simulink model "c8mfpid"  (R2019b)
settings: Solver=VariableStepAuto  StartTime=0.0  StopTime=20  RelTol=1e-11
PreLoadFcn:
  | s=fotf('s'); G=1/(0.8*s^2.2+0.5*s^0.9+1);
  | ww=[1e-4, 1e4]; N=11;
libraries: cstblocks x2
settings Model: Creator=xuedi  LastModifiedBy=xuedi
settings DataIOCC: SaveFormat=Array  ReturnWorkspaceOutputs=off
settings DebuggingCC: UnconnectedInputMsg=none  UnconnectedOutputMsg=none  UnconnectedLineMsg=none  SFMachineParentedDataDiag=error

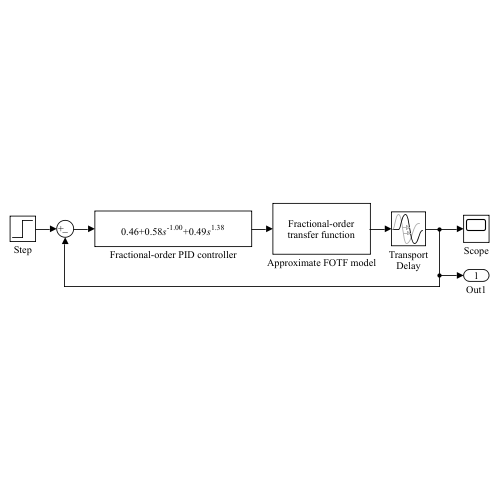
[thumbnail: Simulink's stored preview of the top-level diagram]
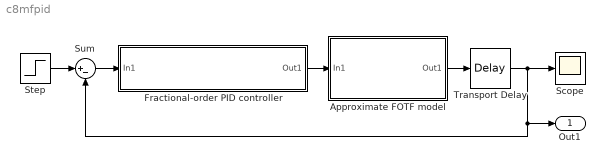
== system c8mfpid ==
  Approximate FOTF model : Subsystem  mask{na=[2.2 0.9 0], a=[0.8 0.5 1], nb=0, b=1, ww=ww, N=N, kFilter=Oustaloup filter, T=0}
      mask prompts: na "Orders of the denominator"; a "Coefficients of the denominator"; nb "Orders of the numerator"; b "Coefficients of the numerator"; ww "Interested frequency range [wb wh]"; N "Filter order"; kFilter "Types of the filter"; T "Delay constant T"
      mask init:
      | if isa(na,'fotf'), G=na; 
      |    else
      |       if length(na)~=length(a)
      |          errordlg('Error','Mismatch on the denominator'), 
      |       end
      |       if length(b)~=length(nb)
      |          errordlg('Error','Mismatch on the numerator'), 
      |       end
      |       G=fotf(a,na,b,nb);
      |    end
      |    switch kFilter
      |       case 1, str='ousta_fod'; 
      |       case 2, str='new_fod'; 
      |       case 3, str='matsude_fod';
      |    end
      |    wb=ww(1); wh=ww(2); G1=high_order(G,str,wb,wh,N); 
      |    G1.ioDelay=T;
      mask TypeOptions kFilter: Oustaloup filter | Modified Oustaloup filter
      mask Display: disp('Fractional-order\ntransfer function')
  Fractional-order PID controller : Subsystem  mask{Kp=0.45966, II=[0.5761 0.99627], DD=[0.49337 1.3792], N=N, ww=ww, kFilter=Oustaloup filter}
      mask prompts: Kp "Proportional Kp"; II "Integral [Ki lam]"; DD "Differentiation [Kd mu]"; N "Filter order"; ww "Interested frequency range [wb wh]"; kFilter "Types of the filter"
      mask init:
      | if isa(Kp,'fotf'), a=Kp;
      |       lam=a.den.na; mu=a.num.na; mu=mu(1)-lam; b=a.num.a; Kd=b(1); Kp=b(2); Ki=b(3);
      |    else, II=[II 1]; DD=[DD 1]; Ki=II(1); lam=II(2); Kd=DD(1); mu=DD(2); end
      |    s=tf('s'); 
      |    sI=ousta_fod(1-lam,N,ww(1),ww(2)); sD=ousta_fod(mu,N,ww(1),ww(2));
      |    Gc=Kp+Ki*sI/s+Kd*sD;
      |    if abs(Ki)>0, sI=[sprintf('%.2f',Ki),'{\its}^{' sprintf('%.2f',-lam), '}']; end
      |    if abs(Kd)>0, sD=[sprintf('%.2f',Kd),'{\its}^{' sprintf('%.2f',mu), '}']; end
      |    str=sprintf('%.2f',Kp);
      |    if abs(Ki)>0, if sI(1)~='-', sI=['+' sI]; end, str=[str,sI]; end
      |    if abs(Kd)>0, if sD(1)~='-', sD=['+' sD]; end, str=[str,sD]; end
      mask TypeOptions kFilter: Oustaloup filter | Modified Oustaloup filter
      mask Display: disp(str,'texmode','on')
  Scope : Scope
  Step : Step  Time=0  SampleTime=0
  Sum : Sum  Inputs=|+-
  Transport Delay : TransportDelay  BufferSize=60000
  Out1 : Outport
  wires:
  Step/1 -> Sum/1
  Sum/1 -> Fractional-order PID controller/1(In1)
  Fractional-order PID controller/1(Out1) -> Approximate FOTF model/1(In1)
  Approximate FOTF model/1(Out1) -> Transport Delay/1
  Transport Delay/1 -> Out1/1, Sum/2, Scope/1

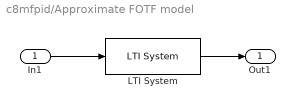
== system c8mfpid/Approximate FOTF model ==
  In1 : Inport
  LTI System : cstblocks/LTI System  sys=G1  IC=[]
  Out1 : Outport
  wires:
  LTI System/1 -> Out1/1
  In1/1 -> LTI System/1

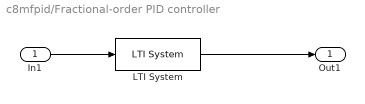
== system c8mfpid/Fractional-order PID controller ==
  In1 : Inport
  LTI System : cstblocks/LTI System  sys=Gc  IC=[]
  Out1 : Outport
  wires:
  In1/1 -> LTI System/1
  LTI System/1 -> Out1/1
